simulink model "motorControl"  (R2019a)
settings: Solver=ode3  StartTime=0.0  StopTime=10  RelTol=1e-3  EnableMultiTasking=on
libraries: simulink x2, legoev3lib x2
settings Model: FPTRunName=Active  ExtModeTrigDuration=2  Creator=jvalencia  LastModifiedBy=jvalencia
settings SolverCC: PositivePriorityOrder=on
settings DataIOCC: LimitDataPoints=on  SaveFormat=Array
settings OptimizationCC: ExpressionDepthLimit=2147483647  LifeSpan=Inf  MaxStackSize=64
settings DebuggingCC: UnderspecifiedInitializationDetection=Classic  MergeDetectMultiDrivingBlocksExec=none  FcnCallInpInsideContextMsg=warning  BusObjectLabelMismatch=error  AllowSymbolicDim=off  StateNameClashWarn=warning  SFUnexpectedBacktrackingDiag=warning  SFNoUnconditionalDefaultTransitionDiag=warning  SFExecutionAtInitializationDiag=none  ArithmeticOperatorsInVariantConditions=warning
settings HardwareCC: ProdBitPerPointer=32  ProdBitPerSizeT=32  ProdBitPerPtrDiffT=32  ProdLargestAtomicInteger=Long  ProdWordSize=32  ProdHWDeviceType=ARM Compatible->ARM 9  UseEmbeddedCoderFeatures=off
settings ModelReferenceCC: PropagateSignalLabelsOutOfModel=off
settings SFSimCC: SimUseLocalCustomCode=off
settings RTWCC: SystemTargetFile=ert.tlc  HardwareBoard=LEGO MINDSTORMS EV3  TemplateMakefile=ert_default_tmf  RTWVerbose=off  RTWUseLocalCustomCode=off  Toolchain=Sourcery G++ Lite v2009q3  BuildConfiguration=Faster Runs
settings CodeAppCC: StateflowObjectComments=on
settings ERTTargetCC: MultiwordLength=2048  ERTCustomFileBanners=off  SupportContinuousTime=on  SupportNonInlinedSFcns=on  RemoveResetFunc=off  SupportVariableSizeSignals=on  ModelStepFunctionPrototypeControlCompliant=off  ConvertIfToSwitch=off  SuppressUnreachableDefaultCases=off
settings ConfigComp: CovMetricSettings=dw  CovHtmlReporting=on  CovSaveCumulativeToWorkspaceVar=on  CovSaveSingleToWorkspaceVar=on  CovExternalEMLEnable=off  CovSFcnEnable=off

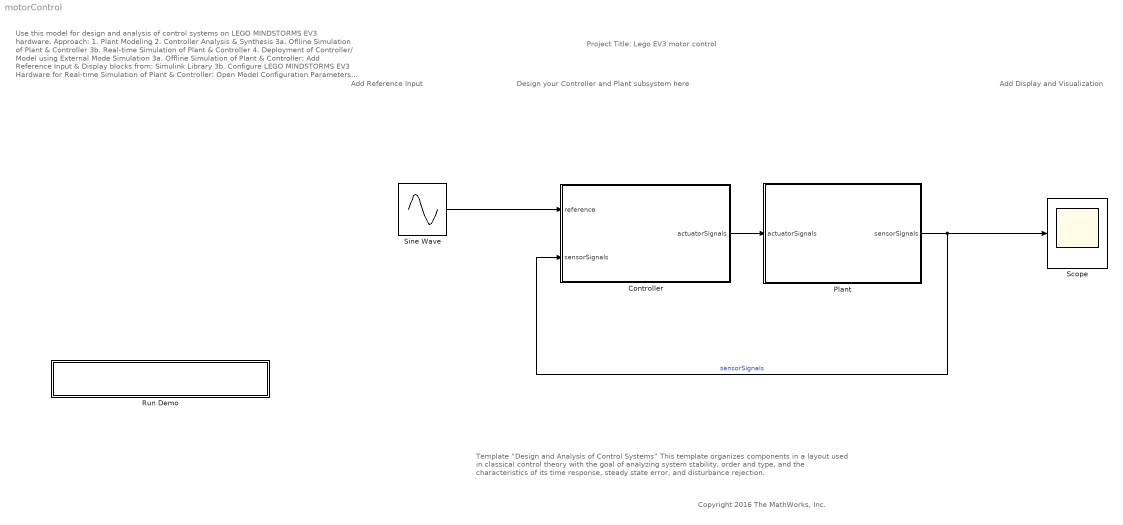
== system motorControl ==
  note: Copyright 2016 The MathWorks, Inc.
  note: Project Title: Lego EV3 motor control
  note: Add Reference Input
  note: Design your Controller and Plant subsystem here
  note: Add Display and Visualization
  note: Template “Design and Analysis of Control Systems” This template organizes components in a layout used in classical control theory with the goal of analyzing system stability, order and type, and the characteristics of its time response, steady state error, and disturbance rejection.
  note: Use this model for design and analysis of control systems on LEGO MINDSTORMS EV3 hardware.
      |
      | Approach:
      |
      | 1. Plant Modeling
      | 2. Controller Analysis & Synthesis
      | 3a. Oflline Simulation of Plant & Controller
      | 3b. Real-time Simulation of Plant & Controller
      | 4. Deployment of Controller/ Model using External Mode
      |
      | Simulation
      |
      | 3a. Offline Simulation of Plant & Controller:
      |
      | Add Reference Input & Display blocks from:
      | Simulink Library
      |
      | 3b. Configure LEGO MINDSTORMS EV3 Hardware for Real-time Simulation of Plant & Controller:
      |
      | Open Model Configuration Parameters dialog
      | Under the Hardware Implementation option, select the desired LEGO MINDSTORMS EV3 hardware from the Hardware bboard parameter list.
      |
      | 4. Deployment of the Model/Controller on LEGO
      | MINDSTORMS EV3 Hardware (External Mode)
      |
      | On the Simulink Editor toolbar, set simulation mode to External
      |
      | External mode will stop when the number of seconds specified in the Simulation stop time parameter elapses.
      |
      | Learn More:
      |
      | Drive with PID Control
  Controller : Subsystem
  Plant : Subsystem
  Run Demo : Subsystem  Description=Controls host-side RTDX processing.
      mask Display: pic=imread('ev3ExternalMode.png');image(pic);
  Scope : Scope
  Sine Wave : Sin  SineType=Sample based  Amplitude=100  SampleTime=0.1
  wires:
  Controller/1(actuatorSignals) -> Plant/1(actuatorSignals)
  Plant/1(sensorSignals) -> Controller/2(sensorSignals), Scope/1  "sensorSignals"
  Sine Wave/1 -> Controller/1(reference)

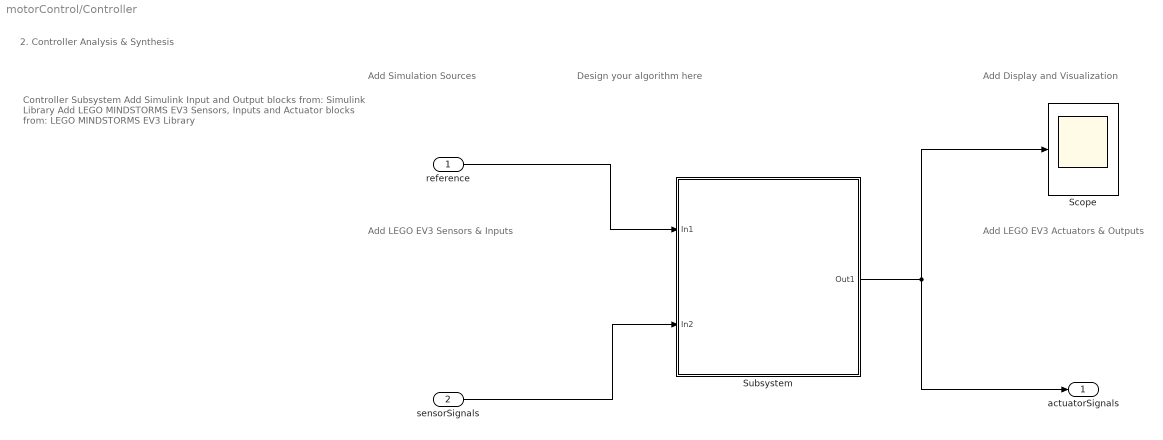
== system motorControl/Controller ==
  note: Add Display and Visualization
  note: Design your algorithm here
  note: Add Simulation Sources
  note: Add LEGO EV3 Sensors & Inputs
  note: Add LEGO EV3 Actuators & Outputs
  note: 2. Controller Analysis & Synthesis
  note: Controller Subsystem
      |
      | Add Simulink Input and Output blocks from:
      | Simulink Library
      | Add LEGO MINDSTORMS EV3 Sensors, Inputs and Actuator blocks from:
      | LEGO MINDSTORMS EV3 Library
  reference : Inport
  sensorSignals : Inport  Port=2
  Scope : Scope
  Subsystem : Subsystem
  actuatorSignals : Outport
  wires:
  sensorSignals/1 -> Subsystem/2(In2)
  Subsystem/1(Out1) -> actuatorSignals/1, Scope/1
  reference/1 -> Subsystem/1(In1)

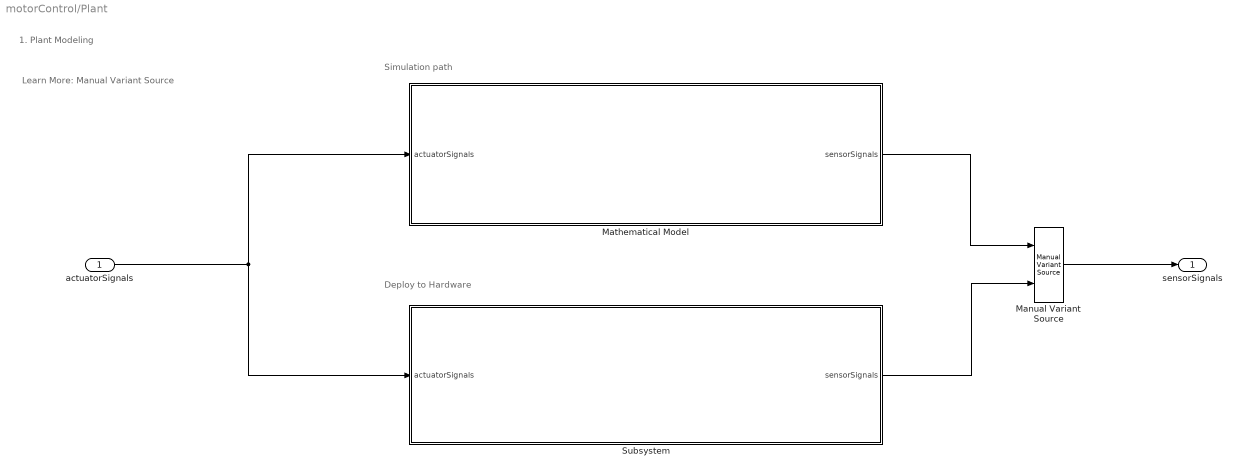
== system motorControl/Plant ==
  note: Deploy to Hardware
  note: Simulation path
  note: 1. Plant Modeling
  note: Learn More:
      |
      | Manual Variant Source
  actuatorSignals : Inport
  Manual Variant Source : simulink/Signal Routing/Manual Variant Source  NumChoices=2  LabelModeActiveChoice=V_1
      settings: SourceProductName=Simulink
  Mathematical Model : Subsystem  VariantControl=plantModel==1
  Subsystem : Subsystem  VariantControl=plantModel==2
  sensorSignals : Outport
  wires:
  actuatorSignals/1 -> Mathematical Model/1(actuatorSignals), Subsystem/1(actuatorSignals)
  Mathematical Model/1(sensorSignals) -> Manual Variant Source/1
  Subsystem/1(sensorSignals) -> Manual Variant Source/2
  Manual Variant Source/1 -> sensorSignals/1

== system motorControl/Run Demo ==

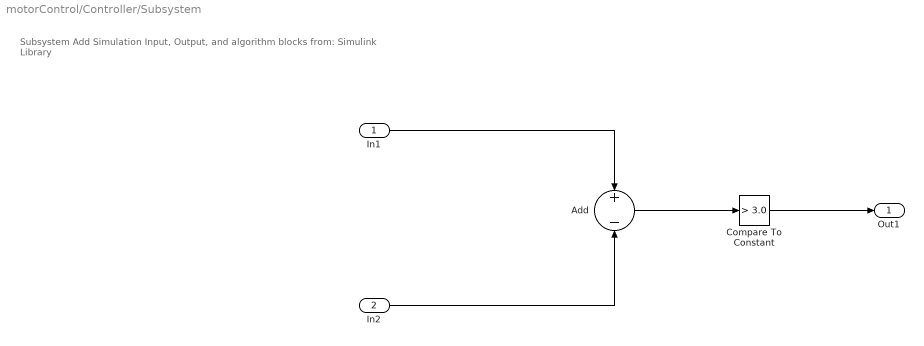
== system motorControl/Controller/Subsystem ==
  note: Subsystem
      |
      | Add Simulation Input, Output, and algorithm blocks from:
      | Simulink Library
  In1 : Inport
  In2 : Inport  Port=2
  Add : Sum  Inputs=+-
  Compare To Constant : simulink/Logic and Bit Operations/Compare To Constant  relop=>  const=3.0  OutDataTypeStr=boolean
  Out1 : Outport
  wires:
  In2/1 -> Add/2
  In1/1 -> Add/1
  Add/1 -> Compare To Constant/1
  Compare To Constant/1 -> Out1/1

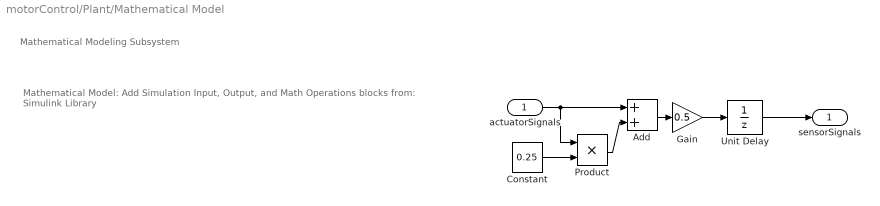
== system motorControl/Plant/Mathematical Model ==
  note: Mathematical Model:
      |
      | Add Simulation Input, Output, and Math Operations blocks from:
      | Simulink Library
  note: Mathematical Modeling Subsystem
  actuatorSignals : Inport
  Add : Sum
  Constant : Constant  Value=0.25  SampleTime=-1
  Gain : Gain  Gain=0.5
  Product : Product
  Unit Delay : UnitDelay  SampleTime=-1  HasFrameUpgradeWarning=on
  sensorSignals : Outport
  wires:
  actuatorSignals/1 -> Product/1, Add/1
  Add/1 -> Gain/1
  Product/1 -> Add/2
  Gain/1 -> Unit Delay/1
  Constant/1 -> Product/2
  Unit Delay/1 -> sensorSignals/1

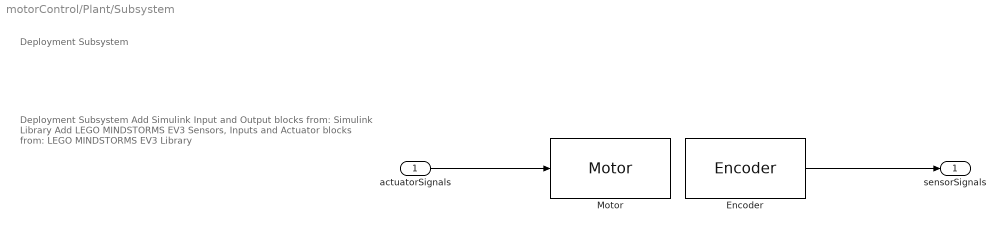
== system motorControl/Plant/Subsystem ==
  note: Deployment Subsystem
      | Add Simulink Input and Output blocks from:
      | Simulink Library
      | Add LEGO MINDSTORMS EV3 Sensors, Inputs and Actuator blocks from:
      | LEGO MINDSTORMS EV3 Library
  note: Deployment Subsystem
  actuatorSignals : Inport
  Encoder : legoev3lib/Encoder  portNumber=A  opMode=No reset  sampleTime=0.1
      settings: SourceProductName=Simulink Support Package for LEGO MINDSTORMS EV3 Hardware  SourceProductBaseCode=LEGOEV3
  Motor : legoev3lib/Motor  sportNumber=A  sstopAction=Brake
  sensorSignals : Outport
  wires:
  actuatorSignals/1 -> Motor/1
  Encoder/1 -> sensorSignals/1
